simulink model "IEEE34bus_v2019b_Phasor_PI_ZIPload"  (R2024a)
settings: Solver=ode4  StartTime=0.0  StopTime=60  FixedStep=Ts  MaxStep=1e-4  RelTol=1e-4
InitFcn:
  | a=1; % Loading Factor
  | Ts=0.1;% For Delay Blocks in Voltage Regulator Controls
  | % phase to sequence conversion of RXB matrices
  | c=1*exp(sqrt(-1)*(120*pi/180));
  | T=[1 1 1;1 c*c c;1 c c*c];
  | Tinv=1/3*[1 1 1;1 c c*c;1 c*c c];
  | 
  | % Simulation data for the IEEE 34 Node Test Feeder model
  | mi2km = 1.60934;%  miles to km conversion
  | ft2km = 0.0003048; % feet to km conversion
  | ms2F = 1*1e-6/(2*pi*60);% microsiemens to Farads conversion
  | 
  | %% Configuration 300 - series reactance - ohm/mile
  | R_300 = [1.3368 0.2101 0.2130;0.2101 1.3238 0.2066;0.2130 0.2066 1.3294];
  | X_300 = [1.3343 0.5779 0.5015;0.5779 1.3569 0.4591;0.5015 0.4591 1.3471];
  | % charging susceptance - microsiemens/mile
  | B_300 = [5.3350 -1.5313 -0.9943;-1.5313 5.0979 -0.6212;-0.9943 -0.6212 4.8880];
  | 
  | R_300 = R_300/mi2km;
  | Rseq=Tinv*R_300*T;
  | R1_300=Rseq(2,2);R0_300=Rseq(1,1);
  | 
  | L_300 = (X_300/(2*pi*60))/mi2km;
  | Lseq=Tinv*L_300*T;
  | L1_300=Lseq(2,2);L0_300=Lseq(1,1);
  | 
  | C_300 =(B_300*ms2F)/mi2km;
  | Cseq=Tinv*C_300*T;
  | C1_300=Cseq(2,2);C0_300=Cseq(1,1);
  | 
  | %% Configuration 301 - series reactance - ohm/mile
  | R_301 = [1.9300 0.2327 0.2359;0.2327 1.9157 0.2288;0.2359 0.2288 1.9219];
  | X_301 = [1.4115 0.6442 0.5691;0.6442 1.4281 0.5238;0.5691 0.5238 1.4209];
  | % charging susceptance - microsiemens/mile
  | B_301 = [5.1207 -1.4364 -0.9402;-1.4364 4.9055 -0.5951;-0.9402 -0.5951 4.7154];
  | 
  | R_301 = R_301/mi2km;
  | Rseq=Tinv*R_301*T;
  | R1_301=Rseq(2,2);R0_301=Rseq(1,1);
  | 
  | L_301 = (X_301/(2*pi*60))/mi2km;
  | Lseq=Tinv*L_301*T;
  | L1_301=Lseq(2,2);L0_301=Lseq(1,1);
  | 
  | C_301 =(B_301*ms2F)/mi2km;
  | Cseq=Tinv*C_301*T;
  | C1_301=Cseq(2,2);C0_301=Cseq(1,1);
  | 
  | %% Configuration 302 - series reactance - ohm/mile
  | R_302 = [2.7995 0 0;0 0 0;0 0 0];
  | X_302 = [1.4855 0 0;0 0 0;0 0 0];
  | % charging susceptance - microsiemens/mile
  | B_302 = [4.2251 0 0;0 0 0;0 0 0];
  | 
  | R_302 = R_302/mi2km;
  | Rseq=Tinv*R_302*T;
  | R1_302=Rseq(2,2);R0_302=Rseq(1,1);
  | 
  | L_302 = (X_302/(2*pi*60))/mi2km;
  | Lseq=Tinv*L_302*T;
  | ... (+41 lines)
undefined symbols (not defined in the file or in its folder): find_system, j, m1, m2, m3, Rcc1, Rcc2, Rcc3
libraries: spsSeriesRLCBranchLib x160, spsGroundLib x106, spsVoltageMeasurementLib x100, spsControlledCurrentSourceLib x94, spsPowerPhasorLib x57, spsThreePhaseVIMeasurementLib x37, spsThreePhasePISectionLineLib x20, spsCurrentMeasurementLib x12, spsOnDelayLib x12, spsPiSectionLineLib x11, spsControlledVoltageSourceLib x6, spsDiscreteVariableTimeDelayLib x6
(part 5 of 8)

== system IEEE34bus_v2019b_Phasor_PI_ZIPload/Regulator 2 ==
  Mux : Mux  Inputs=3
  Single Phase SVR_A : Subsystem  LoadFcn=find_system(gcs,'FollowLinks', 'on', 'LookUnderMasks', 'all');  mask(Single-Phase OLTC){pNom=5e6/3, fNom=60, vNom=24.9e3/sqrt(3), ctRatio=100, ptRatio=120, DeltaU=0.00625, TapMinMax=[-16 16], InitialTap=13, TapSelectionTime=13, RegulatorOn=on, Regulator=[124/120  2/120  2], Comp=[2.5 1.5]}
      mask prompts: pNom "Nominal Power (VA)"; fNom "Nominal Frequency (Hz)"; vNom "Nominal Voltage (Vrms)"; ctRatio "Primary CT Rating (A)"; ptRatio "PT Ratio"; DeltaU "Voltage Step Per Tap (pu)"; TapMinMax "Minimum and Maximum Tap Positions"; InitialTap "Initial Tap Position"; TapSelectionTime "Tap Selection Time (s)"; RegulatorOn "Voltage Regulator"; Regulator "Voltage Regulator [ Vref(pu) DeadBand(pu)  Delay(s)]"; Comp "Compensator Settings [R (V) X(V)]"
      mask help:
      | Models a single-phase On Load Tap Changer (OLTC). The single-phase secondary of multi-tap winding is modeled with a Variable-Ratio Transformer block.
      |
      | The transformer voltage ratio U2/U1 (in pu) is given by:
      |                 U2/U1= 1+TapPosition*DeltaU
      | Tap position 0 corresponds to nominal voltage ratio.
      |
      | When Voltage regulator is 'on',  voltage regulator asks for a tap change if:
      |                  abs(Vm-Vref)>DeadBand/2  during a time  t > Delay.
      |
      | where 'Vm' is voltage measured at regulating point and Vref is reference voltage.
      | With line drop compensation, Vm=Vsec-Isec(R+jX)
      mask init:
      | RegulatorVref=Regulator(1);
      | RegulatorDeadBand=Regulator(2);
      | RegulatorDelay=Regulator(3);
      | Rc=Comp(1);
      | Xc=Comp(2);
      mask TypeOptions RegulatorOn: off | on
      mask Callback RegulatorOn:
      | tempMaskVis=get_param(gcb,'MaskVisibilities');
      | if strcmp(get_param(gcb,'RegulatorOn'),'on')
      | 	tempMaskVis{11}='on';
      | 	set_param(gcb,'MaskVisibilities',tempMaskVis);
      | else
      | 	tempMaskVis{11}='off';
      | 	set_param(gcb,'MaskVisibilities',tempMaskVis);
      | end
      | if strcmp(get_param(gcb,'RegulatorOn'),'on')
      | 	tempMaskVis{12}='on';
      | 	set_param(gcb,'MaskVisibilities',tempMaskVis);
      | else
      | 	tempMaskVis{12}='off';
      | 	set_param(gcb,'MaskVisibilities',tempMaskVis);
      | end
      mask DialogControl Container8 Prompt: Setup
      mask DialogControl Container13 Prompt: Regulator Parameters
      mask Display:
      | color('blue');
      | r=50;x=40;y=80;
      | th = 0:pi/100:2*pi;
      | f = r * exp(j*th) + x+j*y;
      | plot(real(f), imag(f));
      | color('red');
      | plot([-10 90],[30,130])
      | plot([75 90],[125,130])
      | plot([85 90],[115,130])
      | color('black')
      | port_label('Lconn',1,'S');port_label('Rconn',1,'L');
  Single Phase SVR_B : Subsystem  LoadFcn=find_system(gcs,'FollowLinks', 'on', 'LookUnderMasks', 'all');  mask(Single-Phase OLTC){pNom=5e6/3, fNom=60, vNom=24.9e3/sqrt(3), ctRatio=100, ptRatio=120, DeltaU=0.00625, TapMinMax=[-16 16], InitialTap=11, TapSelectionTime=13, RegulatorOn=on, Regulator=[124/120  2/120  2], Comp=[2.5 1.5]}
      mask prompts: pNom "Nominal Power (VA)"; fNom "Nominal Frequency (Hz)"; vNom "Nominal Voltage (Vrms)"; ctRatio "Primary CT Rating (A)"; ptRatio "PT Ratio"; DeltaU "Voltage Step Per Tap (pu)"; TapMinMax "Minimum and Maximum Tap Positions"; InitialTap "Initial Tap Position"; TapSelectionTime "Tap Selection Time (s)"; RegulatorOn "Voltage Regulator"; Regulator "Voltage Regulator [ Vref(pu) DeadBand(pu)  Delay(s)]"; Comp "Compensator Settings [R (V) X(V)]"
      mask help:
      | Models a single-phase On Load Tap Changer (OLTC). The single-phase secondary of multi-tap winding is modeled with a Variable-Ratio Transformer block.
      |
      | The transformer voltage ratio U2/U1 (in pu) is given by:
      |                 U2/U1= 1+TapPosition*DeltaU
      | Tap position 0 corresponds to nominal voltage ratio.
      |
      | When Voltage regulator is 'on',  voltage regulator asks for a tap change if:
      |                  abs(Vm-Vref)>DeadBand/2  during a time  t > Delay.
      |
      | where 'Vm' is voltage measured at regulating point and Vref is reference voltage.
      | With line drop compensation, Vm=Vsec-Isec(R+jX)
      mask init:
      | RegulatorVref=Regulator(1);
      | RegulatorDeadBand=Regulator(2);
      | RegulatorDelay=Regulator(3);
      | Rc=Comp(1);
      | Xc=Comp(2);
      mask TypeOptions RegulatorOn: off | on
      mask Callback RegulatorOn:
      | tempMaskVis=get_param(gcb,'MaskVisibilities');
      | if strcmp(get_param(gcb,'RegulatorOn'),'on')
      | 	tempMaskVis{11}='on';
      | 	set_param(gcb,'MaskVisibilities',tempMaskVis);
      | else
      | 	tempMaskVis{11}='off';
      | 	set_param(gcb,'MaskVisibilities',tempMaskVis);
      | end
      | if strcmp(get_param(gcb,'RegulatorOn'),'on')
      | 	tempMaskVis{12}='on';
      | 	set_param(gcb,'MaskVisibilities',tempMaskVis);
      | else
      | 	tempMaskVis{12}='off';
      | 	set_param(gcb,'MaskVisibilities',tempMaskVis);
      | end
      mask DialogControl Container8 Prompt: Setup
      mask DialogControl Container13 Prompt: Regulator Parameters
      mask Display:
      | color('blue');
      | r=50;x=40;y=80;
      | th = 0:pi/100:2*pi;
      | f = r * exp(j*th) + x+j*y;
      | plot(real(f), imag(f));
      | color('red');
      | plot([-10 90],[30,130])
      | plot([75 90],[125,130])
      | plot([85 90],[115,130])
      | color('black')
      | port_label('Lconn',1,'S');port_label('Rconn',1,'L');
  Single Phase SVR_C : Subsystem  LoadFcn=find_system(gcs,'FollowLinks', 'on', 'LookUnderMasks', 'all');  mask(Single-Phase OLTC){pNom=5e6/3, fNom=60, vNom=24.9e3/sqrt(3), ctRatio=100, ptRatio=120, DeltaU=0.00625, TapMinMax=[-16 16], InitialTap=12, TapSelectionTime=13, RegulatorOn=on, Regulator=[124/120  2/120  2], Comp=[2.5 1.5]}
      mask prompts: pNom "Nominal Power (VA)"; fNom "Nominal Frequency (Hz)"; vNom "Nominal Voltage (Vrms)"; ctRatio "Primary CT Rating (A)"; ptRatio "PT Ratio"; DeltaU "Voltage Step Per Tap (pu)"; TapMinMax "Minimum and Maximum Tap Positions"; InitialTap "Initial Tap Position"; TapSelectionTime "Tap Selection Time (s)"; RegulatorOn "Voltage Regulator"; Regulator "Voltage Regulator [ Vref(pu) DeadBand(pu)  Delay(s)]"; Comp "Compensator Settings [R (V) X(V)]"
      mask help:
      | Models a single-phase On Load Tap Changer (OLTC). The single-phase secondary of multi-tap winding is modeled with a Variable-Ratio Transformer block.
      |
      | The transformer voltage ratio U2/U1 (in pu) is given by:
      |                 U2/U1= 1+TapPosition*DeltaU
      | Tap position 0 corresponds to nominal voltage ratio.
      |
      | When Voltage regulator is 'on',  voltage regulator asks for a tap change if:
      |                  abs(Vm-Vref)>DeadBand/2  during a time  t > Delay.
      |
      | where 'Vm' is voltage measured at regulating point and Vref is reference voltage.
      | With line drop compensation, Vm=Vsec-Isec(R+jX)
      mask init:
      | RegulatorVref=Regulator(1);
      | RegulatorDeadBand=Regulator(2);
      | RegulatorDelay=Regulator(3);
      | Rc=Comp(1);
      | Xc=Comp(2);
      mask TypeOptions RegulatorOn: off | on
      mask Callback RegulatorOn:
      | tempMaskVis=get_param(gcb,'MaskVisibilities');
      | if strcmp(get_param(gcb,'RegulatorOn'),'on')
      | 	tempMaskVis{11}='on';
      | 	set_param(gcb,'MaskVisibilities',tempMaskVis);
      | else
      | 	tempMaskVis{11}='off';
      | 	set_param(gcb,'MaskVisibilities',tempMaskVis);
      | end
      | if strcmp(get_param(gcb,'RegulatorOn'),'on')
      | 	tempMaskVis{12}='on';
      | 	set_param(gcb,'MaskVisibilities',tempMaskVis);
      | else
      | 	tempMaskVis{12}='off';
      | 	set_param(gcb,'MaskVisibilities',tempMaskVis);
      | end
      mask DialogControl Container8 Prompt: Setup
      mask DialogControl Container13 Prompt: Regulator Parameters
      mask Display:
      | color('blue');
      | r=50;x=40;y=80;
      | th = 0:pi/100:2*pi;
      | f = r * exp(j*th) + x+j*y;
      | plot(real(f), imag(f));
      | color('red');
      | plot([-10 90],[30,130])
      | plot([75 90],[125,130])
      | plot([85 90],[115,130])
      | color('black')
      | port_label('Lconn',1,'S');port_label('Rconn',1,'L');
  A : PMIOPort  Side=Left
  a : PMIOPort  Port=2  Side=Right
  B : PMIOPort  Port=3  Side=Left
  b : PMIOPort  Port=4  Side=Right
  C : PMIOPort  Port=5  Side=Left
  c : PMIOPort  Port=6  Side=Right
  Tap : Outport
  wires:
  Mux/1 -> Tap/1
  Single Phase SVR_C/1(Tap) -> Mux/3
  Single Phase SVR_B/1(Tap) -> Mux/2
  Single Phase SVR_A/1(Tap) -> Mux/1
  connections:
  Single Phase SVR_C/RConn1 -- c/RConn1
  Single Phase SVR_C/LConn1 -- C/RConn1
  Single Phase SVR_B/RConn1 -- b/RConn1
  Single Phase SVR_B/LConn1 -- B/RConn1
  Single Phase SVR_A/LConn1 -- A/RConn1
  Single Phase SVR_A/RConn1 -- a/RConn1

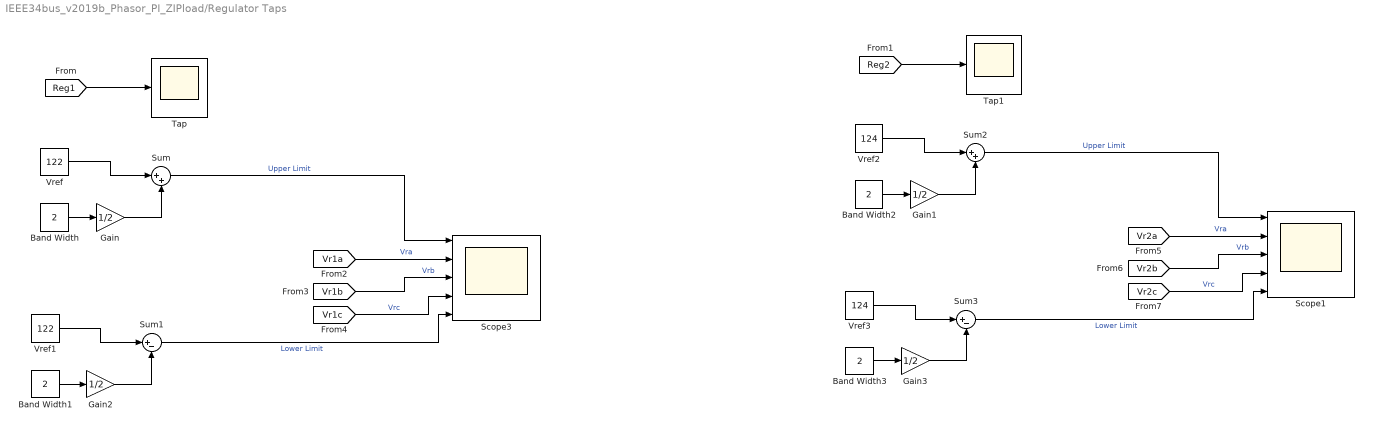
== system IEEE34bus_v2019b_Phasor_PI_ZIPload/Regulator Taps ==
  Band Width{,1..3} (4 alike) : Constant  Value=2
  Gain{,1..3} (4 alike) : Gain  Gain=1/2
  Scope1 : Scope  NumInputPorts=5
  Scope3 : Scope  NumInputPorts=5
  Sum : Sum  Inputs=|++
  Sum1 : Sum  Inputs=|+-
  Sum2 : Sum  Inputs=|++
  Sum3 : Sum  Inputs=|+-
  Tap : Scope
  Tap1 : Scope
  Vref : Constant  Value=122
  Vref1 : Constant  Value=122
  Vref2 : Constant  Value=124
  Vref3 : Constant  Value=124
  wires:
  Vref/1 -> Sum/1
  Gain2/1 -> Sum1/2
  Band Width/1 -> Gain/1
  Gain/1 -> Sum/2
  [Reg1] -> Tap/1
  [Vr1c] -> Scope3/4  "Vrc"
  Band Width1/1 -> Gain2/1
  Sum/1 -> Scope3/1  "Upper Limit"
  Vref1/1 -> Sum1/1
  Sum1/1 -> Scope3/5  "Lower Limit"
  [Vr1b] -> Scope3/3  "Vrb"
  [Vr1a] -> Scope3/2  "Vra"
  [Vr2a] -> Scope1/2  "Vra"
  [Vr2b] -> Scope1/3  "Vrb"
  Sum3/1 -> Scope1/5  "Lower Limit"
  Vref3/1 -> Sum3/1
  Sum2/1 -> Scope1/1  "Upper Limit"
  Band Width3/1 -> Gain3/1
  [Vr2c] -> Scope1/4  "Vrc"
  [Reg2] -> Tap1/1
  Gain1/1 -> Sum2/2
  Band Width2/1 -> Gain1/1
  Gain3/1 -> Sum3/2
  Vref2/1 -> Sum2/1

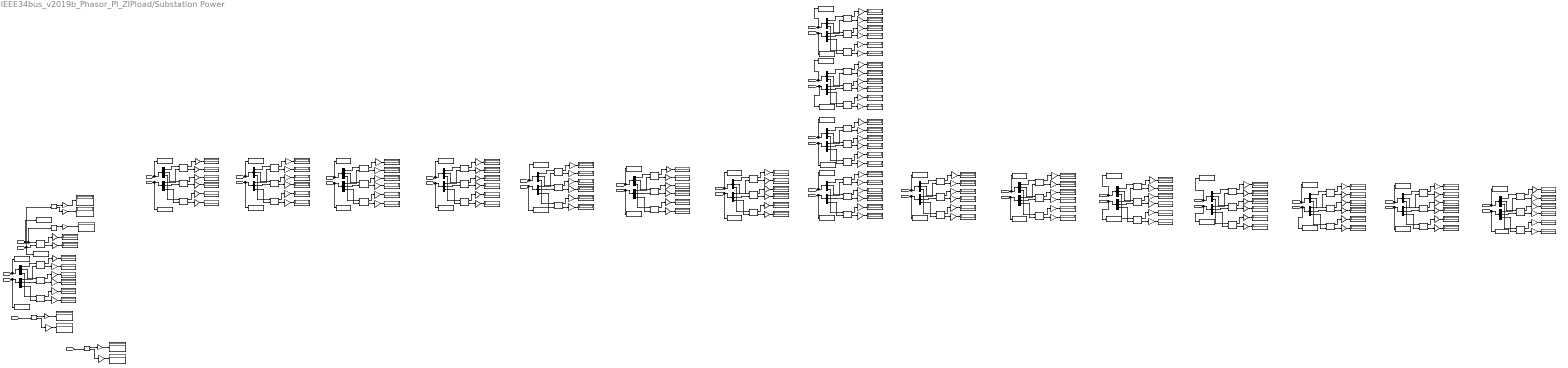
== system IEEE34bus_v2019b_Phasor_PI_ZIPload/Substation Power ==
  note: SYSTEM PHASE PHASE PHASE TOTAL
      | INPUT -------(A)-------|-------(B)-------|-------(C)-------|-------------------
      | kW : 759.136 | 666.663 | 617.072 | 2042.872
      | kVAr : 171.727 | 90.137 | 28.394 | 290.258
  note: PHASE B
  note: PHASE B
  note: PHASE B
  note: PHASE B
  note: PHASE A
  note: PHASE B
  note: PHASE B
  note: PHASE C
  note: TOTAL
  note: PHASE A
  note: PHASE C
  note: PHASE A
  note: PHASE C
  note: PHASE A
  note: PHASE A
  note: PHASE C
  note: PHASE B
  note: PHASE C
  note: PHASE A
  note: PHASE A
  note: PHASE A
  note: PHASE C
  note: PHASE C
  note: PHASE C
  note: PHASE B
  note: PHASE B
  note: PHASE B
  note: PHASE A
  note: PHASE A
  note: PHASE C
  note: PHASE B
  note: PHASE B
  note: PHASE A
  note: PHASE A
  note: PHASE A
  note: PHASE C
  note: PHASE B
  note: PHASE B
  note: PHASE C
  note: PHASE A
  note: Current 800- 802 AMP/DG
      | -------(A)-------|---------(B)----------|-------(C)-------
      | 51.56 -12.74 44.57 -127.70 40.92 117.37
  note: PHASE B
  note: PHASE C
  note: PHASE A
  note: PHASE C
  note: PHASE B
  note: PHASE C
  note: PHASE C
  note: PHASE C
  note: PHASE C
  note: PHASE A
  note: PHASE A
  note: PHASE A
  note: PHASE B
  note: PHASE C
  note: PHASE B
  note: PHASE B
  note: PHASE C
  note: PHASE A
  Complex to Magnitude-Angle{4..7} (4 alike) : ComplexToMagnitudeAngle
  Demux{2..39} (38 alike) : Demux  Outputs=3
  Display{15..137} (123 alike) : Display
  Gain{15..16,22..92,94..126,128..137} (116 alike) : Gain  Gain=1e-3
  Gain127 : Gain  Gain=1/sqrt(2)
  Gain17 : Gain  Gain=180/pi
  Gain18 : Gain  Gain=1/sqrt(2)
  Gain19 : Gain  Gain=180/pi
  Gain20 : Gain  Gain=1/sqrt(2)
  Gain21 : Gain  Gain=180/pi
  Gain93 : Gain  Gain=1/(24900/sqrt(3))*1/sqrt(2)
  "Power (3ph, Phasor)1" : spsPower3phPhasorLib/Power (3ph, Phasor)
      settings: LibrarySourceBlock=|
      | sps_lib/Sensors and Measurements/Power
      | (3ph, Phasor)
  Power (Phasor){3..59} (57 alike) : spsPowerPhasorLib/Power (Phasor)
      settings: LibrarySourceBlock=|
      | sps_lib/Sensors and Measurements/Power
      | (Phasor)
  To Workspace : ToWorkspace  VariableName=V802  SampleTime=-1
      settings: MaxDataPoints=1  Save2DSignal=2-D array (concatenate along first dimension)
  To Workspace1 : ToWorkspace  VariableName=I802  SampleTime=-1
      settings: MaxDataPoints=1  Save2DSignal=2-D array (concatenate along first dimension)
  To Workspace10 : ToWorkspace  VariableName=VRG10  SampleTime=-1
      settings: MaxDataPoints=1  Save2DSignal=2-D array (concatenate along first dimension)
  To Workspace11 : ToWorkspace  VariableName=IRG10  SampleTime=-1
      settings: MaxDataPoints=1  Save2DSignal=2-D array (concatenate along first dimension)
  To Workspace12 : ToWorkspace  VariableName=V850  SampleTime=-1
      settings: MaxDataPoints=1  Save2DSignal=2-D array (concatenate along first dimension)
  To Workspace13 : ToWorkspace  VariableName=I850  SampleTime=-1
      settings: MaxDataPoints=1  Save2DSignal=2-D array (concatenate along first dimension)
  To Workspace14 : ToWorkspace  VariableName=V816  SampleTime=-1
      settings: MaxDataPoints=1  Save2DSignal=2-D array (concatenate along first dimension)
  To Workspace15 : ToWorkspace  VariableName=I816  SampleTime=-1
      settings: MaxDataPoints=1  Save2DSignal=2-D array (concatenate along first dimension)
  To Workspace16 : ToWorkspace  VariableName=V818  SampleTime=-1
      settings: MaxDataPoints=1  Save2DSignal=2-D array (concatenate along first dimension)
  To Workspace17 : ToWorkspace  VariableName=I818  SampleTime=-1
      settings: MaxDataPoints=1  Save2DSignal=2-D array (concatenate along first dimension)
  To Workspace18 : ToWorkspace  VariableName=V820  SampleTime=-1
      settings: MaxDataPoints=1  Save2DSignal=2-D array (concatenate along first dimension)
  To Workspace19 : ToWorkspace  VariableName=I820  SampleTime=-1
      settings: MaxDataPoints=1  Save2DSignal=2-D array (concatenate along first dimension)
  To Workspace2 : ToWorkspace  VariableName=V806  SampleTime=-1
      settings: MaxDataPoints=1  Save2DSignal=2-D array (concatenate along first dimension)
  To Workspace20 : ToWorkspace  VariableName=V822  SampleTime=-1
      settings: MaxDataPoints=1  Save2DSignal=2-D array (concatenate along first dimension)
  To Workspace21 : ToWorkspace  VariableName=I822  SampleTime=-1
      settings: MaxDataPoints=1  Save2DSignal=2-D array (concatenate along first dimension)
  To Workspace22 : ToWorkspace  VariableName=V824  SampleTime=-1
      settings: MaxDataPoints=1  Save2DSignal=2-D array (concatenate along first dimension)
  To Workspace23 : ToWorkspace  VariableName=I824  SampleTime=-1
      settings: MaxDataPoints=1  Save2DSignal=2-D array (concatenate along first dimension)
  To Workspace24 : ToWorkspace  VariableName=V828  SampleTime=-1
      settings: MaxDataPoints=1  Save2DSignal=2-D array (concatenate along first dimension)
  To Workspace25 : ToWorkspace  VariableName=I828  SampleTime=-1
      settings: MaxDataPoints=1  Save2DSignal=2-D array (concatenate along first dimension)
  To Workspace26 : ToWorkspace  VariableName=V830  SampleTime=-1
      settings: MaxDataPoints=1  Save2DSignal=2-D array (concatenate along first dimension)
  To Workspace27 : ToWorkspace  VariableName=I830  SampleTime=-1
      settings: MaxDataPoints=1  Save2DSignal=2-D array (concatenate along first dimension)
  To Workspace28 : ToWorkspace  VariableName=V854  SampleTime=-1
      settings: MaxDataPoints=1  Save2DSignal=2-D array (concatenate along first dimension)
  To Workspace29 : ToWorkspace  VariableName=I854  SampleTime=-1
      settings: MaxDataPoints=1  Save2DSignal=2-D array (concatenate along first dimension)
  To Workspace3 : ToWorkspace  VariableName=I806  SampleTime=-1
      settings: MaxDataPoints=1  Save2DSignal=2-D array (concatenate along first dimension)
  To Workspace30 : ToWorkspace  VariableName=V852  SampleTime=-1
      settings: MaxDataPoints=1  Save2DSignal=2-D array (concatenate along first dimension)
  To Workspace31 : ToWorkspace  VariableName=I852  SampleTime=-1
      settings: MaxDataPoints=1  Save2DSignal=2-D array (concatenate along first dimension)
  To Workspace32 : ToWorkspace  VariableName=VRG11  SampleTime=-1
      settings: MaxDataPoints=1  Save2DSignal=2-D array (concatenate along first dimension)
  To Workspace33 : ToWorkspace  VariableName=IRG11  SampleTime=-1
      settings: MaxDataPoints=1  Save2DSignal=2-D array (concatenate along first dimension)
  To Workspace34 : ToWorkspace  VariableName=V832  SampleTime=-1
      settings: MaxDataPoints=1  Save2DSignal=2-D array (concatenate along first dimension)
  To Workspace35 : ToWorkspace  VariableName=I832  SampleTime=-1
      settings: MaxDataPoints=1  Save2DSignal=2-D array (concatenate along first dimension)
  To Workspace36 : ToWorkspace  VariableName=V  SampleTime=-1
      settings: Save2DSignal=2-D array (concatenate along first dimension)
  To Workspace37 : ToWorkspace  VariableName=I  SampleTime=-1
      settings: Save2DSignal=2-D array (concatenate along first dimension)
  To Workspace38 : ToWorkspace  VariableName=V800  SampleTime=-1
      settings: MaxDataPoints=1  Save2DSignal=2-D array (concatenate along first dimension)
  To Workspace39 : ToWorkspace  VariableName=I800  SampleTime=-1
      settings: MaxDataPoints=1  Save2DSignal=2-D array (concatenate along first dimension)
  To Workspace4 : ToWorkspace  VariableName=V808  SampleTime=-1
      settings: MaxDataPoints=1  Save2DSignal=2-D array (concatenate along first dimension)
  To Workspace5 : ToWorkspace  VariableName=I808  SampleTime=-1
      settings: MaxDataPoints=1  Save2DSignal=2-D array (concatenate along first dimension)
  To Workspace6 : ToWorkspace  VariableName=V812  SampleTime=-1
      settings: MaxDataPoints=1  Save2DSignal=2-D array (concatenate along first dimension)
  To Workspace7 : ToWorkspace  VariableName=I812  SampleTime=-1
      settings: MaxDataPoints=1  Save2DSignal=2-D array (concatenate along first dimension)
  To Workspace8 : ToWorkspace  VariableName=V814  SampleTime=-1
      settings: MaxDataPoints=1  Save2DSignal=2-D array (concatenate along first dimension)
  To Workspace9 : ToWorkspace  VariableName=I814  SampleTime=-1
      settings: MaxDataPoints=1  Save2DSignal=2-D array (concatenate along first dimension)
  wires:
  Gain98/1 -> Display98/1
  [I818] -> To Workspace17/1, Demux33/1
  Power (Phasor)55/2 -> Gain122/1
  Gain40/1 -> Display40/1
  [V816] -> To Workspace14/1, Demux16/1
  Demux13/2 -> Power (Phasor)18/2
  [I822] -> To Workspace21/1, Demux37/1
  Gain76/1 -> Display76/1
  Gain56/1 -> Display56/1
  Power (Phasor)24/2 -> Gain72/1
  Demux4/2 -> Power (Phasor)7/1
  Power (Phasor)49/1 -> Gain109/1
  [V822] -> To Workspace20/1, Demux36/1
  Power (Phasor)47/1 -> Gain137/1
  Power (Phasor)7/2 -> Gain25/1
  Demux36/1 -> Power (Phasor)56/1
  Gain119/1 -> Display119/1
  Power (Phasor)56/2 -> Gain118/1
  Demux8/3 -> Power (Phasor)11/1
  Power (Phasor)25/1 -> Gain73/1
  Gain77/1 -> Display77/1
  Demux36/3 -> Power (Phasor)55/1
  Demux31/3 -> Power (Phasor)46/2
  Demux16/3 -> Power (Phasor)25/1
  Demux36/2 -> Power (Phasor)54/1
  Demux37/2 -> Power (Phasor)54/2
  Gain18/1 -> Display19/1
  [IRG11] -> To Workspace33/1, Demux29/1
  Gain100/1 -> Display100/1
  Power (Phasor)41/2 -> Gain125/1
  Gain130/1 -> Display130/1
  Gain79/1 -> Display79/1
  Power (Phasor)48/2 -> Gain108/1
  Demux37/3 -> Power (Phasor)55/2
  Gain110/1 -> Display110/1
  Gain58/1 -> Display58/1
  Demux26/3 -> Power (Phasor)40/1
  Power (Phasor)56/1 -> Gain117/1
  Power (Phasor)13/1 -> Gain46/1
  Gain118/1 -> Display118/1
  Demux35/1 -> Power (Phasor)53/2
  Power (Phasor)36/2 -> Gain98/1
  Power (Phasor)55/1 -> Gain121/1
  Demux29/3 -> Power (Phasor)43/2
  [I852] -> To Workspace31/1, Demux27/1
  Demux5/3 -> Power (Phasor)8/2
  Gain63/1 -> Display63/1
  Gain105/1 -> Display105/1
  Demux33/3 -> Power (Phasor)49/2
  Power (Phasor)51/2 -> Gain114/1
  Power (Phasor)43/2 -> Gain136/1
  Power (Phasor)51/1 -> Gain113/1
  Power (Phasor)42/1 -> Gain133/1
  Power (Phasor)47/2 -> Gain100/1
  Gain75/1 -> Display75/1
  Demux15/1 -> Power (Phasor)23/2
  Gain109/1 -> Display109/1
  Demux31/1 -> Power (Phasor)47/2
  Power (Phasor)26/2 -> Gain69/1
  Demux34/2 -> Power (Phasor)51/1
  Demux26/1 -> Power (Phasor)41/1
  Demux35/2 -> Power (Phasor)51/2
  Gain115/1 -> Display115/1
  Gain32/1 -> Display32/1
  Gain113/1 -> Display113/1
  Power (Phasor)23/1 -> Gain62/1
  [V818] -> To Workspace16/1, Demux32/1
  Power (Phasor)52/2 -> Gain116/1
  Gain116/1 -> Display116/1
  Gain96/1 -> Display96/1
  Demux15/2 -> Power (Phasor)21/2
  Power (Phasor)9/1 -> Gain29/1
  Power (Phasor)53/1 -> Gain111/1
  Gain129/1 -> Display129/1
  Power (Phasor)39/1 -> Gain126/1
  Demux32/2 -> Power (Phasor)48/1
  Power (Phasor)40/1 -> Gain129/1
  Gain86/1 -> Display86/1
  [I820] -> To Workspace19/1, Demux35/1
  Gain122/1 -> Display122/1
  Power (Phasor)48/1 -> Gain107/1
  [I808] -> To Workspace5/1, Demux9/1
  Power (Phasor)5/1 -> Gain71/1
  Power (Phasor)25/2 -> Gain74/1
  Power (Phasor)53/2 -> Gain112/1
  Gain107/1 -> Display107/1
  Demux7/3 -> Power (Phasor)58/2
  Gain106/1 -> Display106/1
  Gain42/1 -> Display42/1
  Demux33/2 -> Power (Phasor)48/2
  Demux27/2 -> Power (Phasor)39/2
  Power (Phasor)49/2 -> Gain110/1
  Power (Phasor)7/1 -> Gain24/1
  Power (Phasor)46/2 -> Gain104/1
  Gain125/1 -> Display125/1
  Demux30/1 -> Power (Phasor)47/1
  Power (Phasor)18/1 -> Gain57/1
  Power (Phasor)27/2 -> Gain78/1
  Gain117/1 -> Display117/1
  Power (Phasor)6/2 -> Gain23/1
  Gain101/1 -> Display101/1
  Gain103/1 -> Display103/1
  Demux37/1 -> Power (Phasor)56/2
  Gain45/1 -> Display45/1
  Demux20/2 -> Power (Phasor)30/1
  Gain102/1 -> Display102/1
  Gain104/1 -> Display104/1
  Demux21/2 -> Power (Phasor)30/2
  Power (Phasor)45/2 -> Gain102/1
  Power (Phasor)11/2 -> Gain41/1
  Power (Phasor)45/1 -> Gain101/1
  Gain136/1 -> Display136/1
  Gain87/1 -> Display87/1
  Gain126/1 -> Display126/1
  Demux28/3 -> Power (Phasor)43/1
  Gain65/1 -> Display65/1
  Gain114/1 -> Display114/1
  Power (Phasor)33/1 -> Gain90/1
  Demux2/1 -> Power (Phasor)3/1
  [I800] -> To Workspace39/1, Demux3/1
  Power (Phasor)44/1 -> Gain131/1
  Demux12/2 -> Power (Phasor)18/1
  Power (Phasor)31/2 -> Gain87/1
  Power (Phasor)20/1 -> Gain55/1
  [VRG11] -> To Workspace32/1, Demux28/1
  Power (Phasor)16/2 -> Gain54/1
  Demux29/1 -> Power (Phasor)44/2
  Gain135/1 -> Display135/1
  Demux35/3 -> Power (Phasor)52/2
  Gain133/1 -> Display133/1
  Power (Phasor)43/1 -> Gain135/1
  Demux8/2 -> Power (Phasor)10/1
  Gain132/1 -> Display132/1
  [V828] -> To Workspace24/1, Demux20/1
  Demux28/2 -> Power (Phasor)42/1
  Demux28/1 -> Power (Phasor)44/1
  Gain26/1 -> Display26/1
  Gain97/1 -> Display97/1
  [V852] -> To Workspace30/1, Demux26/1
  Demux34/3 -> Power (Phasor)52/1
  Gain128/1 -> Display128/1
  Gain108/1 -> Display108/1
  Power (Phasor)41/1 -> Gain124/1
  Power (Phasor)40/2 -> Gain130/1
  Power (Phasor)31/1 -> Gain86/1
  [V800] -> To Workspace36/1, Complex to Magnitude-Angle4/1, "Power (3ph, Phasor)1"/1
  Demux27/3 -> Power (Phasor)40/2
  Power (Phasor)21/2 -> Gain65/1
  Power (Phasor)4/2 -> Gain60/1
  Demux25/3 -> Power (Phasor)37/2
  Gain134/1 -> Display134/1
  Gain44/1 -> Display44/1
  Demux3/3 -> Power (Phasor)5/2
  Gain124/1 -> Display124/1
  Gain99/1 -> Display99/1
  Demux24/3 -> Power (Phasor)37/1
  Power (Phasor)37/2 -> Gain123/1
  Demux32/3 -> Power (Phasor)49/1
  Gain123/1 -> Display123/1
  Power (Phasor)38/2 -> Gain96/1
  Power (Phasor)37/1 -> Gain99/1
  Power (Phasor)50/1 -> Gain105/1
  Power (Phasor)36/1 -> Gain97/1
  Power (Phasor)34/1 -> Gain92/1
  Demux6/3 -> Power (Phasor)58/1
  Demux24/1 -> Power (Phasor)38/1
  Gain33/1 -> Display33/1
  Power (Phasor)35/1 -> Gain88/1
  Demux20/3 -> Power (Phasor)31/1
  [V830] -> To Workspace26/1, Demux22/1
  Gain74/1 -> Display74/1
  Power (Phasor)46/1 -> Gain103/1
  Power (Phasor)52/1 -> Gain115/1
  Power (Phasor)13/2 -> Gain47/1
  Demux33/1 -> Power (Phasor)50/2
  Gain53/1 -> Display53/1
  Demux14/3 -> Power (Phasor)22/1
  [I830] -> To Workspace27/1, Demux23/1
  Power (Phasor)34/2 -> Gain94/1
  Demux11/3 -> Power (Phasor)16/2
  Gain78/1 -> Display78/1
  Gain89/1 -> Display89/1
  Power (Phasor)30/2 -> Gain85/1
  Demux22/2 -> Power (Phasor)33/1
  Demux22/1 -> Power (Phasor)35/1
  Power (Phasor)35/2 -> Gain89/1
  Power (Phasor)50/2 -> Gain106/1
  Gain88/1 -> Display88/1
  Power (Phasor)33/2 -> Gain91/1
  Demux17/2 -> Power (Phasor)24/2
  Demux22/3 -> Power (Phasor)34/1
  [I814] -> To Workspace9/1, Demux11/1
  Gain94/1 -> Display94/1
  [V824] -> To Workspace22/1, Demux18/1
  Demux23/2 -> Power (Phasor)33/2
  Gain50/1 -> Display50/1
  Demux29/2 -> Power (Phasor)42/2
  Gain91/1 -> Display91/1
  Demux13/3 -> Power (Phasor)19/2
  Gain90/1 -> Display90/1
  Demux23/3 -> Power (Phasor)34/2
  Gain80/1 -> Display80/1
  Demux18/3 -> Power (Phasor)28/1
  Power (Phasor)21/1 -> Gain64/1
  Power (Phasor)30/1 -> Gain84/1
  Demux21/3 -> Power (Phasor)31/2
  [I812] -> To Workspace7/1, Demux39/1
  Demux19/3 -> Power (Phasor)28/2
  Demux39/1 -> Power (Phasor)14/2
  Demux24/2 -> Power (Phasor)36/1
  Demux18/2 -> Power (Phasor)27/1
  Power (Phasor)27/1 -> Gain77/1
  Demux6/2 -> Power (Phasor)57/1
  Gain95/1 -> Display95/1
  Power (Phasor)29/2 -> Gain76/1
  Gain71/1 -> Display71/1
  Demux27/1 -> Power (Phasor)41/2
  Power (Phasor)3/2 -> Gain38/1
  Gain51/1 -> Display51/1
  Power (Phasor)32/1 -> Gain81/1
  [I824] -> To Workspace23/1, Demux19/1
  Demux18/1 -> Power (Phasor)29/1
  Gain73/1 -> Display73/1
  Demux16/1 -> Power (Phasor)26/1
  Gain15/1 -> Display15/1
  Power (Phasor)18/2 -> Gain58/1
  Gain24/1 -> Display24/1
  Complex to Magnitude-Angle5/1 -> Gain127/1
  Demux7/1 -> Power (Phasor)9/2
  Gain121/1 -> Display121/1
  Gain69/1 -> Display69/1
  Demux32/1 -> Power (Phasor)50/1
  Gain70/1 -> Display70/1
  [VRG10] -> To Workspace10/1, Demux12/1
  Gain39/1 -> Display39/1
  Demux8/1 -> Power (Phasor)59/1
  Gain57/1 -> Display57/1
  [I850] -> To Workspace13/1, Demux15/1
  Demux6/1 -> Power (Phasor)9/1
  Demux17/3 -> Power (Phasor)25/2
  Gain66/1 -> Display66/1
  Power (Phasor)22/1 -> Gain66/1
  Power (Phasor)44/2 -> Gain132/1
  Demux17/1 -> Power (Phasor)26/2
  Power (Phasor)23/2 -> Gain63/1
  [V850] -> To Workspace12/1, Demux14/1
  Demux7/2 -> Power (Phasor)57/2
  Demux14/2 -> Power (Phasor)21/1
  Gain62/1 -> Display62/1
  [V820] -> To Workspace18/1, Demux34/1
  Power (Phasor)22/2 -> Gain67/1
  Demux15/3 -> Power (Phasor)22/2
  Power (Phasor)19/1 -> Gain59/1
  Gain16/1 -> Display16/1
  [V802] -> To Workspace/1, Demux4/1
  Power (Phasor)15/1 -> Gain51/1
  Power (Phasor)19/2 -> Gain61/1
  Gain112/1 -> Display112/1
  Gain52/1 -> Display52/1
  Demux23/1 -> Power (Phasor)35/2
  Gain55/1 -> Display55/1
  Power (Phasor)42/2 -> Gain134/1
  Gain61/1 -> Display61/1
  Demux14/1 -> Power (Phasor)23/1
  Power (Phasor)59/1 -> Gain35/1
  Demux10/1 -> Power (Phasor)17/1
  [V812] -> To Workspace6/1, Demux38/1
  Gain54/1 -> Display54/1
  [I802] -> To Workspace1/1, Demux5/1
  [V800] -> To Workspace38/1, Demux2/1
  Gain59/1 -> Display59/1
  Gain64/1 -> Display64/1
  Gain68/1 -> Display68/1
  Gain31/1 -> Display31/1
  [IRG10] -> To Workspace11/1, Demux13/1
  Demux13/1 -> Power (Phasor)20/2
  Power (Phasor)15/2 -> Gain52/1
  Demux12/3 -> Power (Phasor)19/1
  Demux12/1 -> Power (Phasor)20/1
  [V814] -> To Workspace8/1, Demux10/1
  Gain120/1 -> Display120/1
  Power (Phasor)14/1 -> Gain42/1
  Demux5/1 -> Power (Phasor)6/2
  Demux3/1 -> Power (Phasor)3/2
  Gain43/1 -> Display43/1
  Gain82/1 -> Display82/1
  Demux38/1 -> Power (Phasor)14/1
  Demux11/1 -> Power (Phasor)17/2
  Demux10/2 -> Power (Phasor)15/1
  Demux19/2 -> Power (Phasor)27/2
  Power (Phasor)16/1 -> Gain53/1
  Demux39/3 -> Power (Phasor)13/2
  Power (Phasor)17/1 -> Gain48/1
  [V854] -> To Workspace28/1, Demux24/1
  [V806] -> To Workspace2/1, Demux6/1
  Demux4/3 -> Power (Phasor)8/1
  Gain60/1 -> Display60/1
  Demux11/2 -> Power (Phasor)15/2
  Gain21/1 -> Display20/1
  Power (Phasor)39/2 -> Gain128/1
  Gain22/1 -> Display22/1
  Demux25/1 -> Power (Phasor)38/2
  Gain28/1 -> Display28/1
  Complex to Magnitude-Angle6/2 -> Gain19/1
  Gain48/1 -> Display48/1
  Gain20/1 -> Display21/1
  Gain34/1 -> Display34/1
  [V818] -> Complex to Magnitude-Angle7/1
  Power (Phasor)26/1 -> Gain68/1
  Power (Phasor)54/1 -> Gain119/1
  Complex to Magnitude-Angle7/2 -> Gain21/1
  Gain92/1 -> Display92/1
  Complex to Magnitude-Angle6/1 -> Gain18/1
  Power (Phasor)17/2 -> Gain50/1
  Power (Phasor)54/2 -> Gain120/1
  Demux16/2 -> Power (Phasor)24/1
  [I806] -> To Workspace3/1, Demux7/1
  Demux2/2 -> Power (Phasor)4/1
  Power (Phasor)8/1 -> Gain26/1
  Power (Phasor)57/1 -> Gain31/1
  Demux19/1 -> Power (Phasor)29/2
  Gain27/1 -> Display27/1
  Demux10/3 -> Power (Phasor)16/1
  Power (Phasor)3/1 -> Gain27/1
  Power (Phasor)20/2 -> Gain56/1
  Power (Phasor)5/2 -> Gain82/1
  "Power (3ph, Phasor)1"/2 -> Gain16/1
  Power (Phasor)58/2 -> Gain34/1
  Power (Phasor)28/1 -> Gain79/1
  Demux30/2 -> Power (Phasor)45/1
  Power (Phasor)9/2 -> Gain30/1
  Gain25/1 -> Display25/1
  "Power (3ph, Phasor)1"/1 -> Gain15/1
  Power (Phasor)10/2 -> Gain39/1
  Gain35/1 -> Display35/1
  Power (Phasor)12/2 -> Gain45/1
  Demux9/3 -> Power (Phasor)11/2
  [I828] -> To Workspace25/1, Demux21/1
  [I800] -> Complex to Magnitude-Angle6/1
  Demux30/3 -> Power (Phasor)46/1
  Demux9/1 -> Power (Phasor)59/2
  Demux25/2 -> Power (Phasor)36/2
  Demux38/2 -> Power (Phasor)12/1
  Power (Phasor)58/1 -> Gain33/1
  Power (Phasor)38/1 -> Gain95/1
  Power (Phasor)10/1 -> Gain37/1
  Demux3/2 -> Power (Phasor)4/2
  Demux21/1 -> Power (Phasor)32/2
  Gain49/1 -> Display49/1
  Gain30/1 -> Display30/1
  Gain37/1 -> Display37/1
  Demux26/2 -> Power (Phasor)39/1
  Power (Phasor)24/1 -> Gain70/1
  Power (Phasor)11/1 -> Gain40/1
  Power (Phasor)6/1 -> Gain22/1
  Power (Phasor)29/1 -> Gain75/1
  Power (Phasor)57/2 -> Gain32/1
  [I816] -> To Workspace15/1, Demux17/1
  Power (Phasor)4/1 -> Gain49/1
  Gain111/1 -> Display111/1
  Gain29/1 -> Display29/1
  Power (Phasor)59/2 -> Gain36/1
  Gain127/1 -> Display127/1
  Demux31/2 -> Power (Phasor)45/2
  Demux4/1 -> Power (Phasor)6/1
  Gain41/1 -> Display41/1
  Gain93/1 -> Display93/1
  Gain83/1 -> Display83/1
  Gain38/1 -> Display38/1
  [V832] -> To Workspace34/1, Demux30/1
  Gain85/1 -> Display85/1
  Gain46/1 -> Display46/1
  Gain72/1 -> Display72/1
  Gain23/1 -> Display23/1
  Gain17/1 -> Display17/1
  Demux2/3 -> Power (Phasor)5/1
  Gain36/1 -> Display36/1
  Gain81/1 -> Display81/1
  Demux39/2 -> Power (Phasor)12/2
  Gain137/1 -> Display137/1
  Complex to Magnitude-Angle5/2 -> Gain17/1
  Demux38/3 -> Power (Phasor)13/1
  Demux9/2 -> Power (Phasor)10/2
  Gain67/1 -> Display67/1
  [I832] -> To Workspace35/1, Demux31/1
  Gain131/1 -> Display131/1
  [I854] -> To Workspace29/1, Demux25/1
  Power (Phasor)8/2 -> Gain28/1
  Gain47/1 -> Display47/1
  Complex to Magnitude-Angle4/1 -> Gain93/1
  Power (Phasor)28/2 -> Gain80/1
  Demux5/2 -> Power (Phasor)7/2
  Gain84/1 -> Display84/1
  Power (Phasor)14/2 -> Gain43/1
  [V808] -> To Workspace4/1, Demux8/1
  Power (Phasor)12/1 -> Gain44/1
  Demux34/1 -> Power (Phasor)53/1
  Gain19/1 -> Display18/1
  Complex to Magnitude-Angle7/1 -> Gain20/1
  Demux20/1 -> Power (Phasor)32/1
  Power (Phasor)32/2 -> Gain83/1
  [I800] -> Complex to Magnitude-Angle5/1, To Workspace37/1, "Power (3ph, Phasor)1"/2

== system IEEE34bus_v2019b_Phasor_PI_ZIPload/Regulator 1/Single Phase SVR_A ==
  Line Drop Compensator : Subsystem
  Transformer with Taps : Subsystem
  Voltage Regulator Control : Subsystem
  S : PMIOPort  Tag=PMCPort  Side=Left
  L : PMIOPort  Tag=PMCPort  Port=2  Side=Right
  Tap : Outport  VectorParamsAs1DForOutWhenUnconnected=off
  tag scope: Vr1a=global
  wires:
  Line Drop Compensator/1(Vm) -> [Vr1a], Voltage Regulator Control/1(Vm)
  Voltage Regulator Control/1(Tap) -> Transformer with Taps/1(tap), Tap/1
  Transformer with Taps/1(Isec) -> Line Drop Compensator/1(Isec)
  Transformer with Taps/2(Vsec) -> Line Drop Compensator/2(Vsec)
  connections:
  Transformer with Taps/RConn1 -- L/RConn1
  Transformer with Taps/LConn1 -- S/RConn1

== system IEEE34bus_v2019b_Phasor_PI_ZIPload/Regulator 1/Single Phase SVR_B ==
  Line Drop Compensator : Subsystem
  Transformer with Taps : Subsystem
  Voltage Regulator Control : Subsystem
  S : PMIOPort  Tag=PMCPort  Side=Left
  L : PMIOPort  Tag=PMCPort  Port=2  Side=Right
  Tap : Outport  VectorParamsAs1DForOutWhenUnconnected=off
  tag scope: Vr1b=global
  wires:
  Transformer with Taps/2(Vsec) -> Line Drop Compensator/2(Vsec)
  Transformer with Taps/1(Isec) -> Line Drop Compensator/1(Isec)
  Voltage Regulator Control/1(Tap) -> Transformer with Taps/1(tap), Tap/1
  Line Drop Compensator/1(Vm) -> [Vr1b], Voltage Regulator Control/1(Vm)
  connections:
  Transformer with Taps/LConn1 -- S/RConn1
  Transformer with Taps/RConn1 -- L/RConn1

== system IEEE34bus_v2019b_Phasor_PI_ZIPload/Regulator 1/Single Phase SVR_C ==
  Line Drop Compensator : Subsystem
  Transformer with Taps : Subsystem
  Voltage Regulator Control : Subsystem
  S : PMIOPort  Tag=PMCPort  Side=Left
  L : PMIOPort  Tag=PMCPort  Port=2  Side=Right
  Tap : Outport  VectorParamsAs1DForOutWhenUnconnected=off
  tag scope: Vr1c=global
  wires:
  Line Drop Compensator/1(Vm) -> [Vr1c], Voltage Regulator Control/1(Vm)
  Voltage Regulator Control/1(Tap) -> Transformer with Taps/1(tap), Tap/1
  Transformer with Taps/1(Isec) -> Line Drop Compensator/1(Isec)
  Transformer with Taps/2(Vsec) -> Line Drop Compensator/2(Vsec)
  connections:
  Transformer with Taps/RConn1 -- L/RConn1
  Transformer with Taps/LConn1 -- S/RConn1

== system IEEE34bus_v2019b_Phasor_PI_ZIPload/Regulator 2/Single Phase SVR_A ==
  Line Drop Compensator : Subsystem
  Transformer with Taps : Subsystem
  Voltage Regulator Control : Subsystem
  S : PMIOPort  Tag=PMCPort  Side=Left
  L : PMIOPort  Tag=PMCPort  Port=2  Side=Right
  Tap : Outport  VectorParamsAs1DForOutWhenUnconnected=off
  tag scope: Vr2a=global
  wires:
  Line Drop Compensator/1(Vm) -> [Vr2a], Voltage Regulator Control/1(Vm)
  Voltage Regulator Control/1(Tap) -> Transformer with Taps/1(tap), Tap/1
  Transformer with Taps/1(Isec) -> Line Drop Compensator/1(Isec)
  Transformer with Taps/2(Vsec) -> Line Drop Compensator/2(Vsec)
  connections:
  Transformer with Taps/RConn1 -- L/RConn1
  Transformer with Taps/LConn1 -- S/RConn1

== system IEEE34bus_v2019b_Phasor_PI_ZIPload/Regulator 2/Single Phase SVR_B ==
  Line Drop Compensator : Subsystem
  Transformer with Taps : Subsystem
  Voltage Regulator Control : Subsystem
  S : PMIOPort  Tag=PMCPort  Side=Left
  L : PMIOPort  Tag=PMCPort  Port=2  Side=Right
  Tap : Outport  VectorParamsAs1DForOutWhenUnconnected=off
  tag scope: Vr2b=global
  wires:
  Transformer with Taps/2(Vsec) -> Line Drop Compensator/2(Vsec)
  Transformer with Taps/1(Isec) -> Line Drop Compensator/1(Isec)
  Voltage Regulator Control/1(Tap) -> Transformer with Taps/1(tap), Tap/1
  Line Drop Compensator/1(Vm) -> [Vr2b], Voltage Regulator Control/1(Vm)
  connections:
  Transformer with Taps/LConn1 -- S/RConn1
  Transformer with Taps/RConn1 -- L/RConn1

== system IEEE34bus_v2019b_Phasor_PI_ZIPload/Regulator 2/Single Phase SVR_C ==
  Line Drop Compensator : Subsystem
  Transformer with Taps : Subsystem
  Voltage Regulator Control : Subsystem
  S : PMIOPort  Tag=PMCPort  Side=Left
  L : PMIOPort  Tag=PMCPort  Port=2  Side=Right
  Tap : Outport  VectorParamsAs1DForOutWhenUnconnected=off
  tag scope: Vr2c=global
  wires:
  Line Drop Compensator/1(Vm) -> [Vr2c], Voltage Regulator Control/1(Vm)
  Voltage Regulator Control/1(Tap) -> Transformer with Taps/1(tap), Tap/1
  Transformer with Taps/1(Isec) -> Line Drop Compensator/1(Isec)
  Transformer with Taps/2(Vsec) -> Line Drop Compensator/2(Vsec)
  connections:
  Transformer with Taps/RConn1 -- L/RConn1
  Transformer with Taps/LConn1 -- S/RConn1

== system IEEE34bus_v2019b_Phasor_PI_ZIPload/Regulator 1/Single Phase SVR_A/Line Drop Compensator ==
  note: Vm=Vsec-Isec(Rc+jXc)
  Isec : Inport
  Vsec : Inport  Port=2
  Abs1 : Abs  SaturateOnIntegerOverflow=off
  Gain4 : Gain  Gain=1/sqrt(2)
  Gain5 : Gain  Gain=Rc+j*Xc
  Gain6 : Gain  Gain=1/sqrt(2)
  Sum1 : Sum  Inputs=|+-
  Vm : Outport
  wires:
  Abs1/1 -> Vm/1
  Sum1/1 -> Abs1/1
  Isec/1 -> Gain4/1
  Vsec/1 -> Gain6/1
  Gain4/1 -> Gain5/1
  Gain6/1 -> Sum1/1
  Gain5/1 -> Sum1/2

== system IEEE34bus_v2019b_Phasor_PI_ZIPload/Regulator 1/Single Phase SVR_A/Transformer with Taps ==
  note: Isec on CT Ratio base
  note: Vsec on Pt Ratio base
  tap : Inport
  "    " : Gain  Gain=(1/ptRatio)
  " 1" : Gain  Gain=(1/ctRatio)
  CT : spsCurrentMeasurementLib/Current Measurement  PhasorSimulation=on  OutputType=Complex  PSBequivalent=0
  Ground1 : spsGroundLib/Ground  LConnTagsString=a
  Ground2 : spsGroundLib/Ground  LConnTagsString=a
  Ground3 : spsGroundLib/Ground  LConnTagsString=a
  Memory : Memory
  Memory1 : Memory
  PT : spsVoltageMeasurementLib/Voltage Measurement  PhasorSimulation=on  OutputType=Complex  PSBequivalent=0
  Tap Changing Transformer : Subsystem  mask(Tap Changing Transformer){}
      mask help: Implements a Tap changing two-winding ideal transformer with taps at secondary.
      mask Display:
      | A=[-85 -45 -44 -34 -26 -21 -20 -22 -28 -37 -47 -57 -63 -63 -54 -44 -34 -26 -21 -20 -22 -28 -37 -47 -57 -63 -63 -54 -44 -34 -26 -21 -20 -22 -28 -37 -47 -57 -63 -63 -54 -44 -34 -26 -21 -20 -22 -28 -37 -45 -45 -85];
      | B=[-50 -50 -50 -49 -45 -39 -33 -26 -21 -18 -17 -19 -22 -22 -26 -27 -25 -22 -16 -9 -3 2 6 6 4 1 1 -3 -4 -2 2 7 14 20 26 29 30 28 24 24 21 20 21 25 31 37 44 49 50 50 50 50];
      | C=[85 45 44 34 26 21 20 22 28 37 47 57 63 75 63 54 44 34 26 21 20 22 28 37 47 57 63 75 63 54 44 34 26 21 20 22 28 37 47 57 63 75 63 54 44 34 26 21 20 22 28 37 45 45 85];
      | D=[-50 -50 -50 -49 -45 -39 -33 -26 -21 -18 -17 -19 -22 -22 -22 -26 -27 -25 -22 -16 -9 -3 2 6 6 4 1 1 1 -3 -4 -2 2 7 14 20 26 29 30 28 24 24 24 21 20 21 25 31 37 44 49 50 50 50 50];
      | plot(-85,-100,85,100,A,B,C,D);
      | text(-50,-70, '1');text(40,-70, '2');
      | color('green')
      | port_label('Lconn',1,'+');port_label('Rconn',1,'+');
      | color('blue')
      | disp('N')
  L : PMIOPort  Tag=PMCPort  Side=Right
  S : PMIOPort  Port=2  Side=Left
  Isec : Outport
  Vsec : Outport  Port=2
  wires:
  tap/1 -> Tap Changing Transformer/1(Tap)
  Memory/1 -> Isec/1
  Memory1/1 -> Vsec/1
  " 1"/1 -> Memory/1
  CT/1 -> " 1"/1
  PT/1 -> "    "/1
  "    "/1 -> Memory1/1
  connections:
  Tap Changing Transformer/LConn2 -- Ground3/LConn1
  Tap Changing Transformer/LConn1 -- S/RConn1
  Tap Changing Transformer/RConn2 -- Ground2/LConn1
  CT/RConn1 -- L/RConn1
  PT/LConn1 -- CT/LConn1 -- Tap Changing Transformer/RConn1
  PT/LConn2 -- Ground1/LConn1

== system IEEE34bus_v2019b_Phasor_PI_ZIPload/Regulator 1/Single Phase SVR_A/Voltage Regulator Control ==
  Vm : Inport
  Constant : Constant  Value=RegulatorOn
  Tap Changer Control : Subsystem  mask(Tap Changer Control){MinMaxTap=TapMinMax, InitialPosition=InitialTap, MecDelay=TapSelectionTime}
      mask prompts: MinMaxTap "Minimum and maximum tap number [ Min  Max ] :"; InitialPosition "Initial tap position"; MecDelay "Mechanical delay time"
      mask init:
      | if MecDelay<=0,
      | 	MecDelay=1/60;
      | end
  Voltage regulator : Subsystem  mask{Vref=RegulatorVref*120, DeadBand=RegulatorDeadBand*120, TimeDelay=RegulatorDelay}
      mask prompts: Vref "Vref (on 120v base)"; DeadBand "Deadband (on 120v base)"; TimeDelay "Time delay (s)"
  Tap : Outport
  wires:
  Voltage regulator/2(Down) -> Tap Changer Control/2("Down ")
  Tap Changer Control/1(TapNo) -> Tap/1  "Tap"
  Voltage regulator/1(Up) -> Tap Changer Control/1("Up ")
  Tap Changer Control/2(Ready) -> Voltage regulator/2(Ready)
  Constant/1 -> Voltage regulator/3(RegOn)
  Vm/1 -> Voltage regulator/1(Vmes (pu))

== system IEEE34bus_v2019b_Phasor_PI_ZIPload/Regulator 1/Single Phase SVR_B/Line Drop Compensator ==
  note: Vm=Vsec-Isec(Rc+jXc)
  Isec : Inport
  Vsec : Inport  Port=2
  Abs1 : Abs  SaturateOnIntegerOverflow=off
  Gain4 : Gain  Gain=1/sqrt(2)
  Gain5 : Gain  Gain=Rc+j*Xc
  Gain6 : Gain  Gain=1/sqrt(2)
  Sum1 : Sum  Inputs=|+-
  Vm : Outport
  wires:
  Abs1/1 -> Vm/1
  Sum1/1 -> Abs1/1
  Isec/1 -> Gain4/1
  Vsec/1 -> Gain6/1
  Gain4/1 -> Gain5/1
  Gain6/1 -> Sum1/1
  Gain5/1 -> Sum1/2

== system IEEE34bus_v2019b_Phasor_PI_ZIPload/Regulator 1/Single Phase SVR_B/Transformer with Taps ==
  note: Isec on CT Ratio base
  note: Vsec on Pt Ratio base
  tap : Inport
  "    " : Gain  Gain=(1/ptRatio)
  " 1" : Gain  Gain=(1/ctRatio)
  CT : spsCurrentMeasurementLib/Current Measurement  PhasorSimulation=on  OutputType=Complex  PSBequivalent=0
  Ground1 : spsGroundLib/Ground  LConnTagsString=a
  Ground2 : spsGroundLib/Ground  LConnTagsString=a
  Ground3 : spsGroundLib/Ground  LConnTagsString=a
  Memory : Memory
  Memory1 : Memory
  PT : spsVoltageMeasurementLib/Voltage Measurement  PhasorSimulation=on  OutputType=Complex  PSBequivalent=0
  Tap Changing Transformer : Subsystem  mask(Tap Changing Transformer){}
      mask help: Implements a Tap changing two-winding ideal transformer with taps at secondary.
      mask Display:
      | A=[-85 -45 -44 -34 -26 -21 -20 -22 -28 -37 -47 -57 -63 -63 -54 -44 -34 -26 -21 -20 -22 -28 -37 -47 -57 -63 -63 -54 -44 -34 -26 -21 -20 -22 -28 -37 -47 -57 -63 -63 -54 -44 -34 -26 -21 -20 -22 -28 -37 -45 -45 -85];
      | B=[-50 -50 -50 -49 -45 -39 -33 -26 -21 -18 -17 -19 -22 -22 -26 -27 -25 -22 -16 -9 -3 2 6 6 4 1 1 -3 -4 -2 2 7 14 20 26 29 30 28 24 24 21 20 21 25 31 37 44 49 50 50 50 50];
      | C=[85 45 44 34 26 21 20 22 28 37 47 57 63 75 63 54 44 34 26 21 20 22 28 37 47 57 63 75 63 54 44 34 26 21 20 22 28 37 47 57 63 75 63 54 44 34 26 21 20 22 28 37 45 45 85];
      | D=[-50 -50 -50 -49 -45 -39 -33 -26 -21 -18 -17 -19 -22 -22 -22 -26 -27 -25 -22 -16 -9 -3 2 6 6 4 1 1 1 -3 -4 -2 2 7 14 20 26 29 30 28 24 24 24 21 20 21 25 31 37 44 49 50 50 50 50];
      | plot(-85,-100,85,100,A,B,C,D);
      | text(-50,-70, '1');text(40,-70, '2');
      | color('green')
      | port_label('Lconn',1,'+');port_label('Rconn',1,'+');
      | color('blue')
      | disp('N')
  L : PMIOPort  Tag=PMCPort  Side=Right
  S : PMIOPort  Port=2  Side=Left
  Isec : Outport
  Vsec : Outport  Port=2
  wires:
  tap/1 -> Tap Changing Transformer/1(Tap)
  Memory/1 -> Isec/1
  Memory1/1 -> Vsec/1
  " 1"/1 -> Memory/1
  CT/1 -> " 1"/1
  PT/1 -> "    "/1
  "    "/1 -> Memory1/1
  connections:
  Tap Changing Transformer/LConn2 -- Ground3/LConn1
  Tap Changing Transformer/LConn1 -- S/RConn1
  Tap Changing Transformer/RConn2 -- Ground2/LConn1
  CT/RConn1 -- L/RConn1
  PT/LConn1 -- CT/LConn1 -- Tap Changing Transformer/RConn1
  PT/LConn2 -- Ground1/LConn1

== system IEEE34bus_v2019b_Phasor_PI_ZIPload/Regulator 1/Single Phase SVR_B/Voltage Regulator Control ==
  Vm : Inport
  Constant : Constant  Value=RegulatorOn
  Tap Changer Control : Subsystem  mask(Tap Changer Control){MinMaxTap=TapMinMax, InitialPosition=InitialTap, MecDelay=TapSelectionTime}
      mask prompts: MinMaxTap "Minimum and maximum tap number [ Min  Max ] :"; InitialPosition "Initial tap position"; MecDelay "Mechanical delay time"
      mask init:
      | if MecDelay<=0,
      | 	MecDelay=1/60;
      | end
  Voltage regulator : Subsystem  mask{Vref=RegulatorVref*120, DeadBand=RegulatorDeadBand*120, TimeDelay=RegulatorDelay}
      mask prompts: Vref "Vref (on 120v base)"; DeadBand "Deadband (on 120v base)"; TimeDelay "Time delay (s)"
  Tap : Outport
  wires:
  Voltage regulator/2(Down) -> Tap Changer Control/2("Down ")
  Tap Changer Control/1(TapNo) -> Tap/1  "Tap"
  Voltage regulator/1(Up) -> Tap Changer Control/1("Up ")
  Tap Changer Control/2(Ready) -> Voltage regulator/2(Ready)
  Constant/1 -> Voltage regulator/3(RegOn)
  Vm/1 -> Voltage regulator/1(Vmes (pu))

== system IEEE34bus_v2019b_Phasor_PI_ZIPload/Regulator 1/Single Phase SVR_C/Line Drop Compensator ==
  note: Vm=Vsec-Isec(Rc+jXc)
  Isec : Inport
  Vsec : Inport  Port=2
  Abs1 : Abs  SaturateOnIntegerOverflow=off
  Gain4 : Gain  Gain=1/sqrt(2)
  Gain5 : Gain  Gain=Rc+j*Xc
  Gain6 : Gain  Gain=1/sqrt(2)
  Sum1 : Sum  Inputs=|+-
  Vm : Outport
  wires:
  Abs1/1 -> Vm/1
  Sum1/1 -> Abs1/1
  Isec/1 -> Gain4/1
  Vsec/1 -> Gain6/1
  Gain4/1 -> Gain5/1
  Gain6/1 -> Sum1/1
  Gain5/1 -> Sum1/2

== system IEEE34bus_v2019b_Phasor_PI_ZIPload/Regulator 1/Single Phase SVR_C/Transformer with Taps ==
  note: Isec on CT Ratio base
  note: Vsec on Pt Ratio base
  tap : Inport
  "    " : Gain  Gain=(1/ptRatio)
  " 1" : Gain  Gain=(1/ctRatio)
  CT : spsCurrentMeasurementLib/Current Measurement  PhasorSimulation=on  OutputType=Complex  PSBequivalent=0
  Ground1 : spsGroundLib/Ground  LConnTagsString=a
  Ground2 : spsGroundLib/Ground  LConnTagsString=a
  Ground3 : spsGroundLib/Ground  LConnTagsString=a
  Memory : Memory
  Memory1 : Memory
  PT : spsVoltageMeasurementLib/Voltage Measurement  PhasorSimulation=on  OutputType=Complex  PSBequivalent=0
  Tap Changing Transformer : Subsystem  mask(Tap Changing Transformer){}
      mask help: Implements a Tap changing two-winding ideal transformer with taps at secondary.
      mask Display:
      | A=[-85 -45 -44 -34 -26 -21 -20 -22 -28 -37 -47 -57 -63 -63 -54 -44 -34 -26 -21 -20 -22 -28 -37 -47 -57 -63 -63 -54 -44 -34 -26 -21 -20 -22 -28 -37 -47 -57 -63 -63 -54 -44 -34 -26 -21 -20 -22 -28 -37 -45 -45 -85];
      | B=[-50 -50 -50 -49 -45 -39 -33 -26 -21 -18 -17 -19 -22 -22 -26 -27 -25 -22 -16 -9 -3 2 6 6 4 1 1 -3 -4 -2 2 7 14 20 26 29 30 28 24 24 21 20 21 25 31 37 44 49 50 50 50 50];
      | C=[85 45 44 34 26 21 20 22 28 37 47 57 63 75 63 54 44 34 26 21 20 22 28 37 47 57 63 75 63 54 44 34 26 21 20 22 28 37 47 57 63 75 63 54 44 34 26 21 20 22 28 37 45 45 85];
      | D=[-50 -50 -50 -49 -45 -39 -33 -26 -21 -18 -17 -19 -22 -22 -22 -26 -27 -25 -22 -16 -9 -3 2 6 6 4 1 1 1 -3 -4 -2 2 7 14 20 26 29 30 28 24 24 24 21 20 21 25 31 37 44 49 50 50 50 50];
      | plot(-85,-100,85,100,A,B,C,D);
      | text(-50,-70, '1');text(40,-70, '2');
      | color('green')
      | port_label('Lconn',1,'+');port_label('Rconn',1,'+');
      | color('blue')
      | disp('N')
  L : PMIOPort  Tag=PMCPort  Side=Right
  S : PMIOPort  Port=2  Side=Left
  Isec : Outport
  Vsec : Outport  Port=2
  wires:
  tap/1 -> Tap Changing Transformer/1(Tap)
  Memory/1 -> Isec/1
  Memory1/1 -> Vsec/1
  " 1"/1 -> Memory/1
  CT/1 -> " 1"/1
  PT/1 -> "    "/1
  "    "/1 -> Memory1/1
  connections:
  Tap Changing Transformer/LConn2 -- Ground3/LConn1
  Tap Changing Transformer/LConn1 -- S/RConn1
  Tap Changing Transformer/RConn2 -- Ground2/LConn1
  CT/RConn1 -- L/RConn1
  PT/LConn1 -- CT/LConn1 -- Tap Changing Transformer/RConn1
  PT/LConn2 -- Ground1/LConn1
